simulink model "data_acq_passiveV5_test"  (R2016b)
settings: Solver=ode5  StartTime=0.0  StopTime=100  FixedStep=.001  RelTol=1e-3
values from neighbouring files (symbols this model uses):
  offset = [0 0]    [Calibration_Run_Script.m]    (also in DAQ_Run_Script.m; bias.m = signal)
undefined symbols (not defined in the file or in its folder): bit, fdesignblkfcn, gcbh, Standard
libraries: slrtlib x9, slrtsoftinglib x8, canmsglib x7, xpcnilib x3, simulink x2, dspfdesign x2
settings Model: xpc_rtwmakecfg_data=_xpccanac2pci_  SimulationMode=external  ExtModeEnableFloating=off  ExtModeTrigDuration=300000  ExtModeTrigDurationFloating=300  ExtModeArchiveFileName=Test  ExtModeArchiveDirName=C:\Users\1108gotthem\Documents\Gotthelf Summer 2017\MATLAB\Test_Archive  ExtModeAutoIncOneShot=on  ExtModeIncDirWhenArm=on  ExtModeAddSuffixToVar=on  Creator=localadmin  LastModifiedBy=1108gotthem
settings SolverCC: EnableConcurrentExecution=on  AutoInsertRateTranBlk=on
settings DataIOCC: SaveFormat=Structure  SignalLoggingSaveFormat=ModelDataLogs  SaveOutput=off  SignalLogging=off  DSMLogging=off
settings OptimizationCC: BlockReduction=off  OptimizeBlockIOStorage=off  BufferReuse=off  GlobalBufferReuse=off  ExpressionFolding=off  EnableMemcpy=off  ExpressionDepthLimit=2147483647  LocalBlockOutputs=off
settings DebuggingCC: UnderspecifiedInitializationDetection=Classic  MergeDetectMultiDrivingBlocksExec=none  SolverPrmCheckMsg=warning  FcnCallInpInsideContextMsg=warning  StateNameClashWarn=warning  SFUnexpectedBacktrackingDiag=warning  SFNoUnconditionalDefaultTransitionDiag=warning  SFExecutionAtInitializationDiag=none
settings HardwareCC: ProdBitPerPointer=32  ProdBitPerSizeT=32  ProdBitPerPtrDiffT=32  ProdLargestAtomicFloat=None  ProdWordSize=32  ProdLongLongMode=on  ProdHWDeviceType=Generic->32-bit x86 compatible
settings ModelReferenceCC: PropagateSignalLabelsOutOfModel=off
settings RTWCC: SystemTargetFile=slrt.tlc  TemplateMakefile=slrt_default_tmf  Description=Simulink Real-Time  CodeExecutionProfiling=on  CodeProfilingSaveOptions=AllData  RTWCompilerOptimization=on
settings SimulinkRealTimeCC: RL32LogBufSizeModifier=10200000  xPCIRQSourceBoard=Speedgoat_IO331  xPCisModelTimeout=off  xPCModelTimeoutSecs=20
settings ConfigComp: CovMetricSettings=dw  CovHtmlReporting=on  CovSaveCumulativeToWorkspaceVar=on  CovSaveSingleToWorkspaceVar=on  CovExternalEMLEnable=off

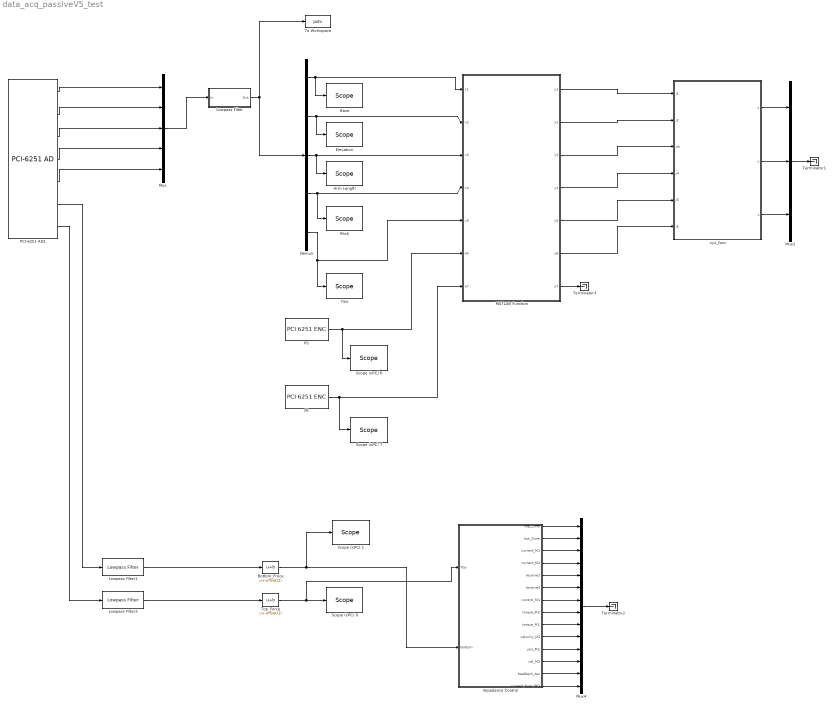
== system data_acq_passiveV5_test ==
  Arm Length : slrtlib/Displays and Logging/Scope   scopeno=3  scopetype=Target  autostart=on  viewmode=Graphical rolling  formatstr='%15.6f'  grid=on  ylimits=[0, 12]  nosamples=15001  noprepostsamples=0  interleave=1  triggermode=FreeRun  triggersignal=1  trigsignalfromport=off  triggerlevel=0.0  triggerslope=Either  triggerscope=1  triggersample=0  filename=data.dat  mode=Lazy  writesize=512  autorestart=off  dynamicfilemode=off  maxwritefilesize=512*1024^2
  Base : slrtlib/Displays and Logging/Scope   scopeno=1  scopetype=Target  autostart=on  viewmode=Graphical rolling  formatstr='%15.6f'  grid=on  ylimits=[0, 12]  nosamples=15001  noprepostsamples=0  interleave=1  triggermode=FreeRun  triggersignal=1  trigsignalfromport=off  triggerlevel=0.0  triggerslope=Either  triggerscope=1  triggersample=0  filename=data.dat  mode=Lazy  writesize=512  autorestart=off  dynamicfilemode=off  maxwritefilesize=512*1024^2
  "Bottom_Froce " : Bias  Bias=-offset(1)
  Demux : Demux  Outputs=5
  Elevation : slrtlib/Displays and Logging/Scope   scopeno=2  scopetype=Target  autostart=on  viewmode=Graphical rolling  formatstr='%15.6f'  grid=on  ylimits=[0, 12]  nosamples=15001  noprepostsamples=0  interleave=1  triggermode=FreeRun  triggersignal=1  trigsignalfromport=off  triggerlevel=0.0  triggerslope=Either  triggerscope=1  triggersample=0  filename=data.dat  mode=Lazy  writesize=512  autorestart=off  dynamicfilemode=off  maxwritefilesize=512*1024^2
  FE : xpcnilib/Incremental Encoder/PCI 6251 ENC   channel=0  countMode=Quadrature Mode x1  initCount=1  reload=off  indexPhase=A low B low  filter=None  sampleTime=0.001  slot=-1
  Impedance Control : Subsystem
  Lowpass Filter : Subsystem  DialogController=fdesignblkfcn  InitFcn=fdesignblkfcn(gcbh, {'InitFcn'});  mask(Lowpass Filter){}
      mask help: Design a lowpass filter
      settings: CopyFcn=fdesignblkfcn(gcbh, {'CopyFcn'});
      mask Help: helpview(mapfilelocation('dsp'), 'dsplowpassfilter');
      mask Display: disp('Lowpass')
  Lowpass Filter1 : dspfdesign/Lowpass Filter  FilterType=FIR  DesignForMinimumOrder=off  FilterOrder=100  PassbandFrequency=5  StopbandFrequency=10  PassbandRipple=1  StopbandAttenuation=60  InheritSampleRate=off  SampleRate=1000  SimulateUsing=Interpreted execution  roundingMode=Floor  coeffsDataTypeStr=fixdt(1,16)
  Lowpass Filter2 : dspfdesign/Lowpass Filter  FilterType=FIR  DesignForMinimumOrder=off  FilterOrder=100  PassbandFrequency=5  StopbandFrequency=10  PassbandRipple=1  StopbandAttenuation=60  InheritSampleRate=off  SampleRate=1000  SimulateUsing=Interpreted execution  roundingMode=Floor  coeffsDataTypeStr=fixdt(1,16)
  MATLAB Function : MATLAB Function  TreatAsAtomicUnit=on
  Mux : Mux  Inputs=5
  Mux2 : Mux  Inputs=3
  Mux4 : Mux  Inputs=14
  PCI-6251 AD1 : xpcnilib/A//D/M Series/PCI-6251 AD  channel=[1,2,3,4,5,7,8]  range=[10,10,10,10,10,10,10]  coupling=[1,1,1,1,1,2,2]  scantime=5e-6  sampletime=0.001  slot=-1
  "PS " : xpcnilib/Incremental Encoder/PCI 6251 ENC   channel=1  countMode=Quadrature Mode x1  initCount=0  reload=off  indexPhase=A low B low  filter=None  sampleTime=0.001  slot=-1
  Pitch : slrtlib/Displays and Logging/Scope   scopeno=4  scopetype=Target  autostart=on  viewmode=Graphical rolling  formatstr='%15.6f'  grid=on  ylimits=[0, 12]  nosamples=15001  noprepostsamples=0  interleave=1  triggermode=FreeRun  triggersignal=1  trigsignalfromport=off  triggerlevel=0.0  triggerslope=Either  triggerscope=1  triggersample=0  filename=data.dat  mode=Lazy  writesize=512  autorestart=off  dynamicfilemode=off  maxwritefilesize=512*1024^2
  Scope (xPC) 1 : slrtlib/Displays and Logging/Scope   scopeno=8  scopetype=Target  autostart=on  viewmode=Graphical rolling  formatstr='%15.6f'  grid=on  ylimits=[-2,2]  nosamples=15001  noprepostsamples=0  interleave=1  triggermode=FreeRun  triggersignal=1  trigsignalfromport=off  triggerlevel=0.0  triggerslope=Either  triggerscope=1  triggersample=0  filename=data.dat  mode=Lazy  writesize=512  autorestart=off  dynamicfilemode=off  maxwritefilesize=512*1024^2
  Scope (xPC) 6 : slrtlib/Displays and Logging/Scope   scopeno=6  scopetype=Target  autostart=on  viewmode=Graphical rolling  formatstr='%15.6f'  grid=on  ylimits=[-15000,15000]  nosamples=15001  noprepostsamples=0  interleave=1  triggermode=FreeRun  triggersignal=1  trigsignalfromport=off  triggerlevel=0.0  triggerslope=Either  triggerscope=1  triggersample=0  filename=data.dat  mode=Lazy  writesize=512  autorestart=off  dynamicfilemode=off  maxwritefilesize=512*1024^2
  Scope (xPC) 7 : slrtlib/Displays and Logging/Scope   scopeno=7  scopetype=Target  autostart=on  viewmode=Graphical rolling  formatstr='%15.6f'  grid=on  ylimits=[-40000,40000]  nosamples=15001  noprepostsamples=0  interleave=1  triggermode=FreeRun  triggersignal=1  trigsignalfromport=off  triggerlevel=0.0  triggerslope=Either  triggerscope=1  triggersample=0  filename=data.dat  mode=Lazy  writesize=512  autorestart=off  dynamicfilemode=off  maxwritefilesize=512*1024^2
  Scope (xPC) 9 : slrtlib/Displays and Logging/Scope   scopeno=9  scopetype=Target  autostart=on  viewmode=Graphical rolling  formatstr='%15.6f'  grid=on  ylimits=[-2,2]  nosamples=15001  noprepostsamples=0  interleave=1  triggermode=FreeRun  triggersignal=1  trigsignalfromport=off  triggerlevel=0.0  triggerslope=Either  triggerscope=1  triggersample=0  filename=data.dat  mode=Lazy  writesize=512  autorestart=off  dynamicfilemode=off  maxwritefilesize=512*1024^2
  Terminator1 : Terminator
  Terminator2 : Terminator
  Terminator3 : Terminator
  To Workspace : ToWorkspace  VariableName=pots  SampleTime=-1
  Top_Force : Bias  Bias=-offset(1)
  Yaw : slrtlib/Displays and Logging/Scope   scopeno=5  scopetype=Target  autostart=on  viewmode=Graphical rolling  formatstr='%15.6f'  grid=on  ylimits=[0, 12]  nosamples=15001  noprepostsamples=0  interleave=1  triggermode=FreeRun  triggersignal=1  trigsignalfromport=off  triggerlevel=0.0  triggerslope=Either  triggerscope=1  triggersample=0  filename=data.dat  mode=Lazy  writesize=512  autorestart=off  dynamicfilemode=off  maxwritefilesize=512*1024^2
  xyz_func : MATLAB Function  TreatAsAtomicUnit=on
  wires:
  PCI-6251 AD1/1 -> Mux/1
  PCI-6251 AD1/2 -> Mux/2
  PCI-6251 AD1/3 -> Mux/3
  PCI-6251 AD1/4 -> Mux/4
  PCI-6251 AD1/5 -> Mux/5
  Demux/2 -> MATLAB Function/2(v2), Elevation/1
  Demux/3 -> MATLAB Function/3(v3), Arm Length/1
  Demux/5 -> MATLAB Function/5(v5), Yaw/1
  PCI-6251 AD1/7 -> Lowpass Filter2/1
  PCI-6251 AD1/6 -> Lowpass Filter1/1
  Demux/1 -> MATLAB Function/1(v1), Base/1
  Mux/1 -> Lowpass Filter/1(In)
  Demux/4 -> MATLAB Function/4(v4), Pitch/1
  MATLAB Function/1(y1) -> xyz_func/1(j1)
  MATLAB Function/2(y2) -> xyz_func/2(j2)
  MATLAB Function/3(y3) -> xyz_func/3(d3)
  MATLAB Function/4(y4) -> xyz_func/4(j4)
  MATLAB Function/5(y5) -> xyz_func/5(j5)
  MATLAB Function/6(y6) -> xyz_func/6(j6)
  xyz_func/1(x) -> Mux2/1
  xyz_func/2(y) -> Mux2/2
  xyz_func/3(z) -> Mux2/3
  "PS "/1 -> MATLAB Function/6(e6), Scope (xPC) 6/1
  Lowpass Filter1/1 -> "Bottom_Froce "/1
  "Bottom_Froce "/1 -> Scope (xPC) 1/1, Impedance Control/2(Bottom)
  Top_Force/1 -> Impedance Control/1(Top), Scope (xPC) 9/1
  Impedance Control/1(top_Zone) -> Mux4/1
  Impedance Control/2(bot_Zone) -> Mux4/2
  Impedance Control/3(current_M1) -> Mux4/3
  Impedance Control/5(receive2) -> Mux4/5
  Impedance Control/6(receive3) -> Mux4/6
  Impedance Control/7(control_M1) -> Mux4/7
  Impedance Control/8(torque_M2) -> Mux4/8
  Impedance Control/9(torque_M1) -> Mux4/9
  Impedance Control/10(velocity_M2) -> Mux4/10
  Impedance Control/11(pos_M2) -> Mux4/11
  Impedance Control/12(vel_M2) -> Mux4/12
  Impedance Control/13(feedback_tau) -> Mux4/13
  Impedance Control/14(current_from_PID) -> Mux4/14
  Lowpass Filter2/1 -> Top_Force/1
  Lowpass Filter/1(Out) -> To Workspace/1, Demux/1
  Impedance Control/4(current_M2) -> Mux4/4
  FE/1 -> MATLAB Function/7(e7), Scope (xPC) 7/1
  Mux4/1 -> Terminator2/1
  Mux2/1 -> Terminator1/1
  MATLAB Function/7(y7) -> Terminator3/1

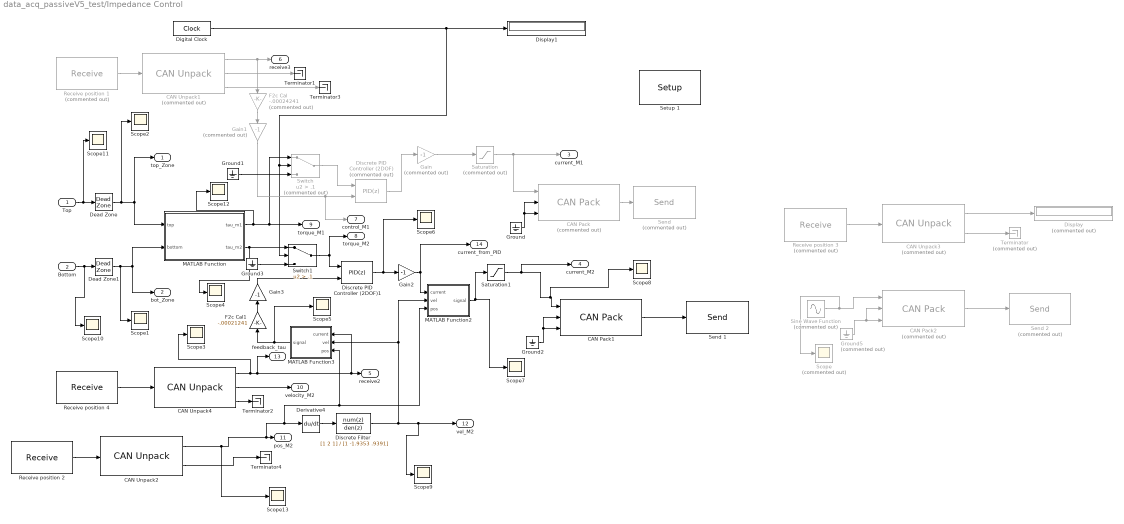
== system data_acq_passiveV5_test/Impedance Control ==
  Top : Inport
  Bottom : Inport  Port=2
  CAN Pack : canmsglib/CAN Pack  Commented=on  MsgList=(none)  MsgName=CAN Msg  MsgIDType=Standard (11-bit identifier)  MsgIdentifier=hex2dec('202')  MsgLength=8  SignalInfo=current$0$16$1$1$1$0$1$0$-Inf$Inf$#null$16$16$1$1$1$0$1$0$-Inf$Inf$#null2$32$32$1$1$1$0$1$0$-Inf$Inf$#  NSignals=3  StartBits=str2num('[int32(0);int32(16);int32(32)]')  SignalSizes=str2num('[int32(16);int32(16);int32(32)]')  ByteOrders=str2num('[int32(1);int32(1);int32(1)]')  DataTypes=str2num('[int32(1);int32(1);int32(1)]')  MultiplexTypes=str2num('[int32(1);int32(1);int32(1)]')  MultiplexValues=str2num('[double(0);double(0);double(0)]')  Factors=str2num('[double(1);double(1);double(1)]')  Offsets=str2num('[double(0);double(0);double(0)]')  Minimums=str2num('[double(-Inf);double(-Inf);double(-Inf)]')  Maximums=str2num('[double(Inf);double(Inf);double(Inf)]')  Remote=off
      settings: DataFormat=manually specified signals
  CAN Pack1 : canmsglib/CAN Pack  MsgList=(none)  MsgName=CAN Msg  MsgIDType=Standard (11-bit identifier)  MsgIdentifier=hex2dec('201')  MsgLength=8  SignalInfo=current$0$16$1$1$1$0$1$0$-Inf$Inf$#null$16$16$1$1$1$0$1$0$-Inf$Inf$#null2$32$32$1$1$1$0$1$0$-Inf$Inf$#  NSignals=3  StartBits=str2num('[int32(0);int32(16);int32(32)]')  SignalSizes=str2num('[int32(16);int32(16);int32(32)]')  ByteOrders=str2num('[int32(1);int32(1);int32(1)]')  DataTypes=str2num('[int32(1);int32(1);int32(1)]')  MultiplexTypes=str2num('[int32(1);int32(1);int32(1)]')  MultiplexValues=str2num('[double(0);double(0);double(0)]')  Factors=str2num('[double(1);double(1);double(1)]')  Offsets=str2num('[double(0);double(0);double(0)]')  Minimums=str2num('[double(-Inf);double(-Inf);double(-Inf)]')  Maximums=str2num('[double(Inf);double(Inf);double(Inf)]')  Remote=off
      settings: DataFormat=manually specified signals
  CAN Pack2 : canmsglib/CAN Pack  Commented=on  MsgList=(none)  MsgName=CAN Msg  MsgIDType=Standard (11-bit identifier)  MsgIdentifier=hex2dec('201')  MsgLength=8  SignalInfo=current$0$16$1$1$1$0$1$0$-Inf$Inf$#null$16$16$1$1$1$0$1$0$-Inf$Inf$#null2$32$32$1$1$1$0$1$0$-Inf$Inf$#  NSignals=3  StartBits=str2num('[int32(0);int32(16);int32(32)]')  SignalSizes=str2num('[int32(16);int32(16);int32(32)]')  ByteOrders=str2num('[int32(1);int32(1);int32(1)]')  DataTypes=str2num('[int32(1);int32(1);int32(1)]')  MultiplexTypes=str2num('[int32(1);int32(1);int32(1)]')  MultiplexValues=str2num('[double(0);double(0);double(0)]')  Factors=str2num('[double(1);double(1);double(1)]')  Offsets=str2num('[double(0);double(0);double(0)]')  Minimums=str2num('[double(-Inf);double(-Inf);double(-Inf)]')  Maximums=str2num('[double(Inf);double(Inf);double(Inf)]')  Remote=off
      settings: DataFormat=manually specified signals
  CAN Unpack1 : canmsglib/CAN Unpack  Commented=on  MsgList=(none)  MsgName=CAN Msg  MsgIDType=Standard (11-bit identifier)  MsgIdentifier=hex2dec('182')  MsgLength=8  SignalInfo=Current$0$16$1$1$1$0$1$0$-Inf$Inf$#null$16$32$1$2$1$0$1$0$-Inf$Inf$#null2$48$16$1$1$1$0$1$0$-Inf$Inf$#  NSignals=3  IDPort=off  TimestampPort=off  ErrorPort=off  RemotePort=off  LengthPort=off  StatusPort=off  StartBits=str2num('[int32(0);int32(16);int32(48)]')  SignalSizes=str2num('[int32(16);int32(32);int32(16)]')  ByteOrders=str2num('[int32(1);int32(1);int32(1)]')  DataTypes=str2num('[int32(1);int32(2);int32(1)]')  MultiplexTypes=str2num('[int32(1);int32(1);int32(1)]')  MultiplexValues=str2num('[double(0);double(0);double(0)]')  Factors=str2num('[double(1);double(1);double(1)]')  Offsets=str2num('[double(0);double(0);double(0)]')  Minimums=str2num('[double(-Inf);double(-Inf);double(-Inf)]')  Maximums=str2num('[double(Inf);double(Inf);double(Inf)]')
  CAN Unpack2 : canmsglib/CAN Unpack  MsgList=(none)  MsgName=CAN Msg  MsgIDType=Standard (11-bit identifier)  MsgIdentifier=hex2dec('281')  MsgLength=8  SignalInfo=pos$0$32$1$1$1$0$1$0$-Inf$Inf$#null$32$32$1$2$1$0$1$0$-Inf$Inf$#  NSignals=2  IDPort=off  TimestampPort=off  ErrorPort=off  RemotePort=off  LengthPort=off  StatusPort=off  StartBits=str2num('[int32(0);int32(32)]')  SignalSizes=str2num('[int32(32);int32(32)]')  ByteOrders=str2num('[int32(1);int32(1)]')  DataTypes=str2num('[int32(1);int32(2)]')  MultiplexTypes=str2num('[int32(1);int32(1)]')  MultiplexValues=str2num('[double(0);double(0)]')  Factors=str2num('[double(1);double(1)]')  Offsets=str2num('[double(0);double(0)]')  Minimums=str2num('[double(-Inf);double(-Inf)]')  Maximums=str2num('[double(Inf);double(Inf)]')
  CAN Unpack3 : canmsglib/CAN Unpack  Commented=on  MsgList=(none)  MsgName=CAN Msg  MsgIDType=Standard (11-bit identifier)  MsgIdentifier=hex2dec('181')  MsgLength=8  SignalInfo=position$0$32$1$1$1$0$1$0$-Inf$Inf$#null$32$32$1$2$1$0$1$0$-Inf$Inf$#  NSignals=2  IDPort=off  TimestampPort=off  ErrorPort=off  RemotePort=off  LengthPort=off  StatusPort=off  StartBits=str2num('[int32(0);int32(32)]')  SignalSizes=str2num('[int32(32);int32(32)]')  ByteOrders=str2num('[int32(1);int32(1)]')  DataTypes=str2num('[int32(1);int32(2)]')  MultiplexTypes=str2num('[int32(1);int32(1)]')  MultiplexValues=str2num('[double(0);double(0)]')  Factors=str2num('[double(1);double(1)]')  Offsets=str2num('[double(0);double(0)]')  Minimums=str2num('[double(-Inf);double(-Inf)]')  Maximums=str2num('[double(Inf);double(Inf)]')
  CAN Unpack4 : canmsglib/CAN Unpack  MsgList=(none)  MsgName=CAN Msg  MsgIDType=Standard (11-bit identifier)  MsgIdentifier=hex2dec('181')  MsgLength=8  SignalInfo=Current$0$16$1$1$1$0$1$0$-Inf$Inf$#vel$16$32$1$2$1$0$1$0$-Inf$Inf$#null$48$16$1$1$1$0$1$0$-Inf$Inf$#  NSignals=3  IDPort=off  TimestampPort=off  ErrorPort=off  RemotePort=off  LengthPort=off  StatusPort=off  StartBits=str2num('[int32(0);int32(16);int32(48)]')  SignalSizes=str2num('[int32(16);int32(32);int32(16)]')  ByteOrders=str2num('[int32(1);int32(1);int32(1)]')  DataTypes=str2num('[int32(1);int32(2);int32(1)]')  MultiplexTypes=str2num('[int32(1);int32(1);int32(1)]')  MultiplexValues=str2num('[double(0);double(0);double(0)]')  Factors=str2num('[double(1);double(1);double(1)]')  Offsets=str2num('[double(0);double(0);double(0)]')  Minimums=str2num('[double(-Inf);double(-Inf);double(-Inf)]')  Maximums=str2num('[double(Inf);double(Inf);double(Inf)]')
  Dead Zone : DeadZone  LowerValue=-.05  UpperValue=.05  SaturateOnIntegerOverflow=on
  Dead Zone1 : DeadZone  LowerValue=-.05  UpperValue=.05  SaturateOnIntegerOverflow=on
  Derivative4 : Derivative
  Digital Clock : DigitalClock  SampleTime=.001
  Discrete Filter : DiscreteFilter  Numerator=[1 2 1]  Denominator=[1 -1.9353 .9391]
  Discrete PID Controller (2DOF) : simulink/Continuous/PID Controller (2DOF)  Commented=on  Controller=PID  TimeDomain=Discrete-time  SampleTime=-1  IntegratorMethod=Forward Euler  FilterMethod=Forward Euler  Form=Parallel  UseFilter=on  ControllerParametersSource=internal  P=-206.434175056882  I=-412868.350113764  D=0  N=100  b=1  c=1  InitialConditionSource=internal  InitialConditionForIntegrator=0  InitialConditionForFilter=0  ExternalReset=none  LimitOutput=off  UpperSaturationLimit=inf  LowerSaturationLimit=-inf  LinearizeAsGain=off  AntiWindupMode=none  Kb=1  TrackingMode=off  Kt=1  PParamMin=[]  PParamMax=[]  IParamMin=[]  IParamMax=[]  DParamMin=[]  DParamMax=[]  NParamMin=[]  NParamMax=[]  bParamMin=[]  bParamMax=[]  cParamMin=[]  cParamMax=[]  KbParamMin=[]  KbParamMax=[]  KtParamMin=[]  KtParamMax=[]  POutMin=[]  POutMax=[]  IOutMin=[]  IOutMax=[]  DOutMin=[]  DOutMax=[]  NOutMin=[]  NOutMax=[]  bOutMin=[]  bOutMax=[]  cOutMin=[]  cOutMax=[]  KbOutMin=[]  KbOutMax=[]  KtOutMin=[]  KtOutMax=[]  IntegratorOutMin=[]  IntegratorOutMax=[]  FilterOutMin=[]  FilterOutMax=[]  SumOutMin=[]  SumOutMax=[]  Sum1OutMin=[]  Sum1OutMax=[]  Sum2OutMin=[]  Sum2OutMax=[]  Sum3OutMin=[]  Sum3OutMax=[]  SumI1OutMin=[]  SumI1OutMax=[]  SumI2OutMin=[]  SumI2OutMax=[]  SumI3OutMin=[]  SumI3OutMax=[]  SumDOutMin=[]  SumDOutMax=[]  SaturationOutMin=[]  SaturationOutMax=[]  IntegratorContinuousStateAttributes=''  IntegratorStateMustResolveToSignalObject=off  IntegratorRTWStateStorageClass=Auto  FilterContinuousStateAttributes=''  FilterStateMustResolveToSignalObject=off  FilterRTWStateStorageClass=Auto  DifferentiatorICPrevScaledInput=0  DifferentiatorOutMin=[]  DifferentiatorOutMax=[]
  Discrete PID Controller (2DOF)1 : simulink/Continuous/PID Controller (2DOF)  Controller=PID  TimeDomain=Discrete-time  SampleTime=-1  IntegratorMethod=Forward Euler  FilterMethod=Forward Euler  Form=Parallel  UseFilter=on  ControllerParametersSource=internal  P=-235.590171722324  I=-471180.343444648  D=0  N=100  b=1  c=1  InitialConditionSource=internal  InitialConditionForIntegrator=0  InitialConditionForFilter=0  ExternalReset=none  LimitOutput=off  UpperSaturationLimit=inf  LowerSaturationLimit=-inf  LinearizeAsGain=off  AntiWindupMode=none  Kb=1  TrackingMode=off  Kt=1  PParamMin=[]  PParamMax=[]  IParamMin=[]  IParamMax=[]  DParamMin=[]  DParamMax=[]  NParamMin=[]  NParamMax=[]  bParamMin=[]  bParamMax=[]  cParamMin=[]  cParamMax=[]  KbParamMin=[]  KbParamMax=[]  KtParamMin=[]  KtParamMax=[]  POutMin=[]  POutMax=[]  IOutMin=[]  IOutMax=[]  DOutMin=[]  DOutMax=[]  NOutMin=[]  NOutMax=[]  bOutMin=[]  bOutMax=[]  cOutMin=[]  cOutMax=[]  KbOutMin=[]  KbOutMax=[]  KtOutMin=[]  KtOutMax=[]  IntegratorOutMin=[]  IntegratorOutMax=[]  FilterOutMin=[]  FilterOutMax=[]  SumOutMin=[]  SumOutMax=[]  Sum1OutMin=[]  Sum1OutMax=[]  Sum2OutMin=[]  Sum2OutMax=[]  Sum3OutMin=[]  Sum3OutMax=[]  SumI1OutMin=[]  SumI1OutMax=[]  SumI2OutMin=[]  SumI2OutMax=[]  SumI3OutMin=[]  SumI3OutMax=[]  SumDOutMin=[]  SumDOutMax=[]  SaturationOutMin=[]  SaturationOutMax=[]  IntegratorContinuousStateAttributes=''  IntegratorStateMustResolveToSignalObject=off  IntegratorRTWStateStorageClass=Auto  FilterContinuousStateAttributes=''  FilterStateMustResolveToSignalObject=off  FilterRTWStateStorageClass=Auto  DifferentiatorICPrevScaledInput=0  DifferentiatorOutMin=[]  DifferentiatorOutMax=[]
  Display : Display  Commented=on
      settings: Format=hex (Stored Integer)
  Display1 : Display
      settings: Format=hex (Stored Integer)
  F2c Cal : Gain  Commented=on  Gain=-.00024241
  F2c Cal1 : Gain  Gain=-.00021241
  Gain : Gain  Commented=on  Gain=-1
  Gain1 : Gain  Commented=on  Gain=-1
  Gain2 : Gain  Gain=-1
  Gain3 : Gain  Gain=-1
  Ground{,1..3} (4 alike) : Ground
  Ground5 : Ground  Commented=on
  MATLAB Function : MATLAB Function  TreatAsAtomicUnit=on
  MATLAB Function2 : MATLAB Function  TreatAsAtomicUnit=on
  MATLAB Function3 : MATLAB Function  TreatAsAtomicUnit=on
  Receive position 1 : slrtsoftinglib/CAN-AC2-PCI SJA 1000/Receive   Commented=on  board=1  canPort=CAN 1  range=Standard (11-bit)  ids=hex2dec('182')  lengths=8  output=CAN_MESSAGE data type  inten=off  ts=0.001  ididx=[1]
  Receive position 2 : slrtsoftinglib/CAN-AC2-PCI SJA 1000/Receive   board=1  canPort=CAN 1  range=Standard (11-bit)  ids=hex2dec('281')  lengths=8  output=CAN_MESSAGE data type  inten=off  ts=0.001  ididx=[1]
  Receive position 3 : slrtsoftinglib/CAN-AC2-PCI SJA 1000/Receive   Commented=on  board=1  canPort=CAN 1  range=Standard (11-bit)  ids=hex2dec('181')  lengths=8  output=CAN_MESSAGE data type  inten=off  ts=0.001  ididx=[0]
  Receive position 4 : slrtsoftinglib/CAN-AC2-PCI SJA 1000/Receive   board=1  canPort=CAN 1  range=Standard (11-bit)  ids=hex2dec('181')  lengths=8  output=CAN_MESSAGE data type  inten=off  ts=0.001  ididx=[0]
  Saturation : Saturate  Commented=on  UpperLimit=1700  LowerLimit=-1700  LinearizeAsGain=off
  Saturation1 : Saturate  UpperLimit=1700  LowerLimit=-1700  LinearizeAsGain=off
  Scope : Scope  Commented=on
  Scope{1..13} (13 alike) : Scope
  "Send " : slrtsoftinglib/CAN-AC2-PCI SJA 1000/Send   Commented=on  board=1  canPort=CAN 1  range=Standard (11-bit)  ids=hex2dec('202')  sizes=[8]  output=off  ts=0.001  ididx=[2]
  Send 1 : slrtsoftinglib/CAN-AC2-PCI SJA 1000/Send   board=1  canPort=CAN 1  range=Standard (11-bit)  ids=hex2dec('201')  sizes=8  output=off  ts=0.001  ididx=[1]
  Send 2 : slrtsoftinglib/CAN-AC2-PCI SJA 1000/Send   Commented=on  board=1  canPort=CAN 1  range=Standard (11-bit)  ids=hex2dec('201')  sizes=8  output=off  ts=0.001  ididx=[1]
  Setup 1 : slrtsoftinglib/CAN-AC2-PCI SJA 1000/Setup   board=1  can1bus=Highspeed (ISO 11898)  can1Baudrate=1 MBaud  can1UserBR=[1,1,4,3]  can2bus=Highspeed (ISO 11898)  can2Baudrate=1 MBaud  can2UserBR=[1,1,4,3]  init=pdo_start  term=pdo_stop  bus_off_out=off  bus_off_rec=Off  ioBaseAddress=-1
  Sine Wave Function : Sin  Commented=on  Amplitude=600  SampleTime=.001
  Switch : Switch  Commented=on  Criteria=u2 > Threshold  Threshold=.1
  Switch1 : Switch  Criteria=u2 > Threshold  Threshold=.1
  Terminator : Terminator  Commented=on
  Terminator{1..4} (4 alike) : Terminator
  top_Zone : Outport
  bot_Zone : Outport  Port=2
  current_M1 : Outport  Port=3
  current_M2 : Outport  Port=4
  receive2 : Outport  Port=5
  receive3 : Outport  Port=6
  control_M1 : Outport  Port=7
  torque_M2 : Outport  Port=8
  torque_M1 : Outport  Port=9
  velocity_M2 : Outport  Port=10
  pos_M2 : Outport  Port=11
  vel_M2 : Outport  Port=12
  feedback_tau : Outport  Port=13
  current_from_PID : Outport  Port=14
  wires:
  Ground/1 -> CAN Pack/2, CAN Pack/3
  CAN Pack/1 -> "Send "/1
  CAN Unpack4/2 -> velocity_M2/1
  Digital Clock/1 -> Display1/1, Switch1/2, Switch/2
  Dead Zone/1 -> Scope2/1, MATLAB Function/1(top), top_Zone/1
  Dead Zone1/1 -> Scope1/1, bot_Zone/1, MATLAB Function/2(bottom)
  Ground2/1 -> CAN Pack1/3, CAN Pack1/2
  MATLAB Function/2(tau_m2) -> Switch1/1, Scope4/1
  CAN Unpack1/1 -> F2c Cal/1, receive3/1
  CAN Unpack1/2 -> Terminator1/1
  Receive position 1/1 -> CAN Unpack1/1
  CAN Unpack1/3 -> Terminator3/1
  CAN Unpack4/3 -> Terminator2/1
  Top/1 -> Scope11/1, Dead Zone/1
  Bottom/1 -> Scope10/1, Dead Zone1/1
  MATLAB Function/1(tau_m1) -> Scope12/1, Switch/1, torque_M1/1
  Discrete PID Controller (2DOF)/1 -> Gain/1
  Discrete PID Controller (2DOF)1/1 -> Scope6/1, Gain2/1
  F2c Cal/1 -> Gain1/1
  F2c Cal1/1 -> Gain3/1
  Gain/1 -> Saturation/1
  Gain1/1 -> control_M1/1, Discrete PID Controller (2DOF)/2
  Gain3/1 -> Discrete PID Controller (2DOF)1/2
  Receive position 2/1 -> CAN Unpack2/1
  CAN Unpack2/2 -> Terminator4/1
  Derivative4/1 -> Discrete Filter/1
  Discrete Filter/1 -> MATLAB Function3/2(vel), MATLAB Function2/2(vel), Scope9/1, vel_M2/1
  Saturation/1 -> current_M1/1, CAN Pack/1
  Ground1/1 -> Switch/3
  Switch/1 -> Discrete PID Controller (2DOF)/1
  Switch1/1 -> torque_M2/1, Discrete PID Controller (2DOF)1/1
  Ground3/1 -> Switch1/3
  CAN Unpack2/1 -> Scope13/1, MATLAB Function3/3(pos), MATLAB Function2/3(pos), Derivative4/1, pos_M2/1
  MATLAB Function3/1(signal) -> Scope5/1, F2c Cal1/1
  MATLAB Function2/1(signal) -> Scope7/1, Saturation1/1
  Gain2/1 -> MATLAB Function2/1(current), current_from_PID/1
  Receive position 3/1 -> CAN Unpack3/1
  CAN Unpack3/1 -> Display/1
  CAN Pack2/1 -> Send 2/1
  Ground5/1 -> CAN Pack2/2, CAN Pack2/3
  CAN Unpack3/2 -> Terminator/1
  Sine Wave Function/1 -> Scope/1, CAN Pack2/1
  CAN Pack1/1 -> Send 1/1
  Receive position 4/1 -> CAN Unpack4/1
  Saturation1/1 -> Scope8/1, CAN Pack1/1, current_M2/1
  CAN Unpack4/1 -> Scope3/1, feedback_tau/1, MATLAB Function3/1(current), receive2/1

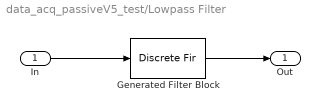
== system data_acq_passiveV5_test/Lowpass Filter ==
  In : Inport
  Generated Filter Block : DiscreteFir  Tag=BlockMethodSubSystem  Coefficients=[-0.00052324228244352597 -5.6057008840111622e-05 -5.9029960060090123e-05 -6.2089092415703651e-05 -6.5235172106602808e-05 -6.8468792239146433e-05 -7.1791170876184978e-05 -7.5199394031231657e-05 -7.8693485466635764e-05 -8.2278777605507031e-05 -8.595347305185517e-05 -8.9721309412065051e-05 -9.3578658035005043e-05 -9.7527959693077641e-05 -0.00010156823183841502 -0.00010570306844346472 -0.0001099328592674625 -0.00011425592773425428 -0.00011867203248127299 -0.0001231799968737532 -0.00012778728307383345 -0.00013249067611977418 -0.00013729314500949554 -0.00014218232070427767 -0.00014716926331734948 -0.00015225602378782298 -0.00015743218992457042 -0.00016269728987213943 -0.00016806238974750827 -0.00017352033232048865 -0.0001790541571821037 -0.00018469470695856038 -0.00019040984292100611 -0.00019621615780973255 -0.00020210453549572777 -0.00020807769136475324 -0.00021413162898923835 -0.00022026741549891577 -0.00022648545623399775 -0.00023278305632693007 -0.00023916116470940019 -0.00024561752902621861 -0.00025215563189431487 -0.00025877239732060919 -0.00026546870783869639 -0.00027224140486980879 -0.00027909126326666029 -0.00028601702953346975 -0.00029301423418495693 -0.0003000833632016655 -0.00030721562663037119 -0.00031442057334346384 -0.00032166470362155413 -0.0003289859106662829 -0.00033634358815721359 -0.00034374313095350431 -0.00035119427093453651 -0.00035868375459999696 -0.0003662039702031097 -0.00037376552352817309 -0.0003813735840803234 -0.00038901495643876518 -0.00039669544877577199 -0.00040441363753715757 -0.00041217530568567532 -0.00041997236920575794 -0.00042779681226945903 -0.00043563648316667354 -0.00044348025734073965 -0.00045131682050124572 -0.00045913146718169523 -0.00046691658695320793 -0.00047466786789203153 -0.00048240036364918733 -0.00049013557695491749 -0.00049790927995173621 -0.00050574222671454687 -0.00051362605492419008 -0.00052149568150616993 -0.00052920115935022743 -0.00053654954320442034 -0.00054357771054403859 -0.00055214790105943346 -0.00055916535223403136 -0.00056666427607138812 -0.00057404465564137052 -0.00058135307459826859 -0.00058858746107408311 -0.00059574654644921473 -0.00060282347017059977 -0.00060981028743565169 -0.00061670493558216505 -0.00062349928924097396 -0.000630192055063267 -0.00063677471765257723 -0.00064324342516180089 -0.00064958972288984044 -0.00065581029697547931 -0.0006619013208642088 -0.00066785686227762093 -0.00067367026968544099 -0.00067932944837409447 -0.00068483347458354069 -0.00069017350542580796 -0.00069535230042428028 -0.00070034879032750846 -0.00070516462522351693 -0.00070979980509052972 -0.00071424020173444002 -0.00071847608015420902 -0.00072251270665083943 -0.00072634337800568096 -0.00072994321245200037 -0.00073333574344273337 -0.00073649156348525686 -0.00073941703893840895 -0.00074210053887124113 -0.00074453916177031048 -0.00074672281031526401 -0.00074864519360783878 -0.00075030132489939145 -0.00075168278519708134 -0.00075278399298329122 -0.00075359502155582811 -0.00075411336084044384 -0.00075433142515719212 -0.00075424619678480674 -0.00075384983500808959 -0.00075313851527801946 -0.0007521083156189119 -0.0007507511200035438 -0.00074906499149087695 -0.00074703433019716707 -0.00074467569886822607 -0.00074193430250794738 -0.00073886247530116969 -0.00073541239059260954 -0.00073157897963701992 -0.0007273769919590344 -0.00072279421000670443 -0.00071781259232127099 -0.00071243669254971711 -0.00070667704483942564 -0.00070052009746154594 -0.00069396076402879247 -0.00068698617116579529 -0.00067959495504656586 -0.00067177723621101009 -0.00066352416222824231 -0.0006548251523169538 -0.00064567650220373897 -0.00063608395400448962 -0.00062605373231083893 -0.00061559312159697338 -0.00060469234669886644 -0.00059333532482305806 -0.00058149012821433687 -0.00056914033755682623 -0.00055628848147566494 -0.00054297275957292416 -0.00052924873470221775 -0.00051510617355876131 -0.0005003889172763155 -0.00048493969539900724 -0.00046944146128394216 -0.00045313869696779349 -0.0004364405176052949 ...(+12253 chars)]
  Out : Outport
  wires:
  In/1 -> Generated Filter Block/1
  Generated Filter Block/1 -> Out/1

== matlab function data_acq_passiveV5_test/xyz_func ==
  data: x output; j1 input; y output; j2 input; d3 input; j4 input; j5 input; j6 input; z output
function [x,y,z] = fcn(j1,j2,d3,j4,j5,j6)
%#codegen

d1=336.55;
%a2=434.46; %original distance from x2 to x4 when arm is fully retracted
a2=406.4; %new distance from x2 to x4 when arm is fully retracted
d4=45.86;
a5=120.51;
d6=67.08;
a6=39.52;

s1=sind(j1);
c1=cosd(j1);
s2=sind(j2);
c2=cosd(j2);
s4=sind(j4);
c4=cosd(j4);
s5=sind(j5);
c5=cosd(j5);
s6=sind(j6);
c6=cosd(j6);

x = -a6*c6*((c1*s2*c5)+s5*((s1*c4)-(c1*c2*s4)))+a6*s6*((s1*s4)+(c1*c2*c4))-d6*((c1*s2*s5)-c5*((s1*c4)-(c1*c2*s4)))-(a5*c1*s2*c5)-a5*s5*((s1*c4)-(c1*c2*s4))-(d4*c1*s2)+((a2+d3)*c1*c2);
y = -a6*c6*((s1*s2*c5)-s5*((c1*c4)+(s1*c2*s4)))-a6*s6*((c1*s4)-(s1*c2*c4))-d6*((s1*s2*s5)+c5*((c1*c4)+(s1*c2*s4)))-(a5*s1*s2*c5)+a5*s5*((c1*c4)+(s1*c2*s4))-(d4*s1*s2)+((a2+d3)*s1*c2);
z = -a6*c6*((c2*c5)+(s2*s4*s5))-(a6*s2*c4*s6)-d6*((c2*s5)-(s2*s4*c5))-(a5*c2*c5)-(a5*s2*s4*s5)-(d4*c2)-((a2+d3)*s2)+d1;

== matlab function data_acq_passiveV5_test/MATLAB Function ==
  data: v1 input; y1 output; v2 input; v3 input; v4 input; v5 input; e6 input; e7 input; y2 output; y3 output; y4 output; y5 output; y6 output; y7 output
function [y1,y2,y3,y4,y5,y6,y7] = volt2deg(v1,v2,v3,v4,v5,e6,e7)
%#codegen

%Enter Calibration Voltages
joint1_zero=7.3609;
joint1_25=8.0502;
joint2=4.353;
joint3_extended=6.6944;
joint3_retracted=0.36547;
joint4=8.8793;
joint5=5.6408;
%-----------------------------------------------
slope1245=(joint1_25 - joint1_zero)/25;
%slope3=(joint3_extended - joint3_retracted)/438; %original
slope3=(joint3_extended - joint3_retracted)/436.56; %new travel

joint1_os=joint1_zero;
%joint2_os=joint2 + (slope1245 * 5.6932); %original
joint2_os=joint2 + (slope1245 * 3.8); %new angle
joint4_os=joint4;
joint5_os=joint5;

y1=(joint1_os - v1)./slope1245;
y2=(joint2_os - v2)./slope1245;
y3=(v3 - joint3_retracted)./slope3;
y4=(v4 - joint4_os)./slope1245;
y5=(v5 - joint5_os)./slope1245;
y6=(pi/180)*(30/18750).*e6;
y7=(pi/180)*(30/33920).*e7;

== matlab function data_acq_passiveV5_test/Impedance Control/MATLAB Function ==
  data: tau_m1 output; top input; tau_m2 output; bottom input
function [tau_m1,tau_m2] = f2t(top,bottom)
%#codegen

F1=(top/1901)*(50/.02)*4.4482216;
F2=(bottom/1901)*(50/.02)*4.4482216;

%Revision 8/12/14
F1ps=(F1/2.7)-(F2/1.588);
F1fe=(F1+F2)/1.588;
F2ps=(-F1/2.7)+(F2/1.588);
F2fe=(F1+F2)/2.7;

Ffe=((10*F1fe)+(17*F2fe))/27;
Fps=(F1ps-F2ps)/2;

tau_m1=Fps*.0435;
tau_m2=Ffe*.065;

end

== matlab function data_acq_passiveV5_test/Impedance Control/MATLAB Function2 ==
  data: current input; vel input; pos input; signal output
function signal = fcn(current,vel,pos)
%#codegen

% y=exp(-pos.^2/15000);
y=1;
z=1;

if vel >= 3e7
    y=1./(1+exp(-.00000004*vel+4));
elseif vel < -3e7
    y=1./(1+exp(.00000002*vel+3.5));
elseif vel < 3e7 && vel >= -3e7
    y=.05;
end

iscale=current.*y;

if pos >= 0
    z=.9./(1+exp(.0002*pos-8));
elseif pos < 0
    z=.9./(1+exp(-.0002*pos-8));
end

signal=iscale.*z;

end

== matlab function data_acq_passiveV5_test/Impedance Control/MATLAB Function3 ==
  data: current input; vel input; signal output; pos input
function signal = fcn(current,vel,pos)
%#codegen

% y=exp(-pos.^2/15000);
y=1;
z=1;

if vel >= 3e7
    y=1./(1+exp(-.00000004*vel+4));
elseif vel < -3e7
    y=1./(1+exp(.00000002*vel+3.5));
elseif vel < 3e7 && vel >= -3e7
    y=.05;
end

iscale=current./y;

if pos >= 0
    z=.9./(1+exp(.0002*pos-8));
elseif pos < 0
    z=.9./(1+exp(-.0002*pos-8));
end

signal=iscale./z;

end
